simulink model "simulation_model"  (R2018b)
settings: Solver=ode45  StartTime=0.0  StopTime=20000  RelTol=1e-3
values from neighbouring files (symbols this model uses):
  DP = polyfit(CL_uav,CD_uav,2)    [intialize.m]
  Dprop = 0.482    [intialize.m]
  J = xlsread('UAVdata.xlsx','P3:P16')    [intialize.m]
  p0 = 0.03840634    [intialize.m]
  p1 = 0.04503419    [intialize.m]
  p2 = -0.06173971    [intialize.m]
  p3 = -0.06297906    [intialize.m]
  Sref = 0.6    [intialize.m]
  xx = [1000 1173.46938776 1346.93877551 1520.40816327 1693.87755102 1867.34693878 2040.81632653 2214.28571429 2387.75510204 2561.2244898 2734.69387755 2908.16326531 ... (50 elements, 1x50)]    [engine_data.mat]
  yy = [1.39285714286 1.7055393586 2.01822157434 2.33090379009 2.64358600583 2.95626822157 3.26895043732 3.58163265306 3.8943148688 4.20699708455 4.51967930029 4.83236151603 ... (50 elements, 1x50)]    [engine_data.mat]
  Zeng = [1318.54879102 1244.05943439 1169.57007776 1095.08072113 1020.59136451 950.389908425 918.779557259 887.169206094 855.558854928 823.948503763 795.179532477 777.776080712 ... (2500 elements, 50x50)]    [engine_data.mat]
settings Model: Creator=Rohith  LastModifiedBy=Rohith

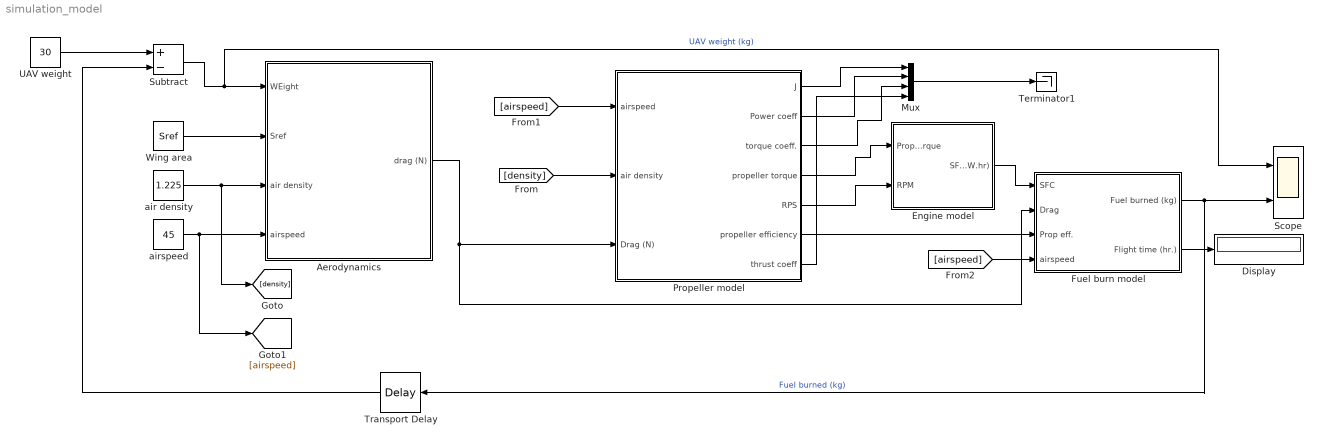
== system simulation_model ==
  Aerodynamics : Subsystem
  Display : Display
  Engine model : Subsystem
  Fuel burn model : Subsystem
  Mux : Mux
  Propeller model : Subsystem
  Scope : Scope  NumInputPorts=2
  Subtract : Sum  Inputs=+-
  Terminator1 : Terminator
  Transport Delay : TransportDelay  DelayTime=0.1
  UAV weight : Constant  Value=30
  Wing area : Constant  Value=Sref
  air density : Constant  Value=1.225
  airspeed : Constant  Value=45
  wires:
  Subtract/1 -> Scope/1, Aerodynamics/1(WEight)  "UAV weight (kg)"
  Wing area/1 -> Aerodynamics/2(Sref)
  air density/1 -> [density], Aerodynamics/3(air density)
  airspeed/1 -> [airspeed], Aerodynamics/4(airspeed)
  Aerodynamics/1(drag (N)) -> Propeller model/3(Drag (N)), Fuel burn model/2(Drag)
  [density] -> Propeller model/2(air density)
  [airspeed] -> Propeller model/1(airspeed)
  Propeller model/4(propeller torque) -> Engine model/1(Prop torque)
  Propeller model/5(RPS) -> Engine model/2(RPM)
  Engine model/1(SFC (kg/W.hr)) -> Fuel burn model/1(SFC)
  [airspeed] -> Fuel burn model/4(airspeed)
  Propeller model/6("propeller efficiency ") -> Fuel burn model/3(Prop eff.)
  Fuel burn model/1(Fuel burned (kg)) -> Scope/2, Transport Delay/1  "Fuel burned (kg)"
  Propeller model/1(J) -> Mux/1
  Propeller model/2(Power coeff) -> Mux/2
  Mux/1 -> Terminator1/1
  Propeller model/3(torque coeff.) -> Mux/3
  Propeller model/7(thrust coeff) -> Mux/4
  Fuel burn model/2(Flight time (hr.)) -> Display/1
  UAV weight/1 -> Subtract/1
  Transport Delay/1 -> Subtract/2

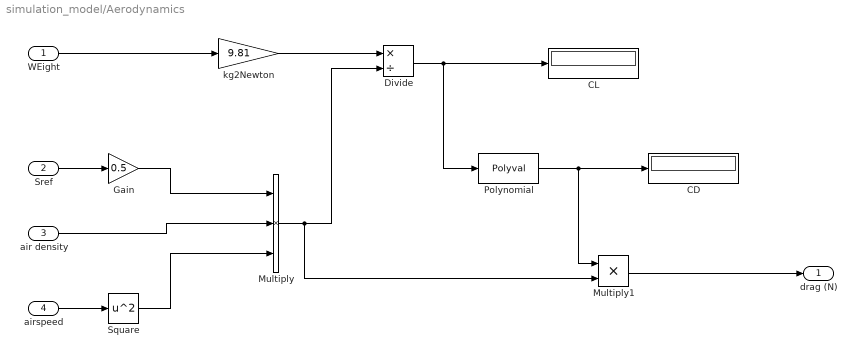
== system simulation_model/Aerodynamics ==
  WEight : Inport
  Sref : Inport  Port=2
  air density : Inport  Port=3
  airspeed : Inport  Port=4
  CD : Display
  CL : Display
  Divide : Product  Inputs=*/
  Gain : Gain  Gain=0.5
  Multiply : Product  Inputs=3
  Multiply1 : Product
  Polynomial : Polyval  Coefs="[DP(1)  DP(2)  DP(3)]"
  Square : Math  Operator=square  SaturateOnIntegerOverflow=on
  kg2Newton : Gain  Gain=9.81
  drag (N) : Outport
  wires:
  Sref/1 -> Gain/1
  Divide/1 -> Polynomial/1, CL/1
  Multiply1/1 -> drag (N)/1
  Square/1 -> Multiply/3
  Polynomial/1 -> Multiply1/1, CD/1
  kg2Newton/1 -> Divide/1
  Gain/1 -> Multiply/1
  Multiply/1 -> Multiply1/2, Divide/2
  WEight/1 -> kg2Newton/1
  airspeed/1 -> Square/1
  air density/1 -> Multiply/2

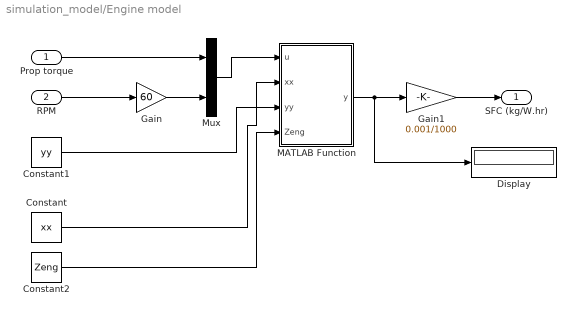
== system simulation_model/Engine model ==
  Prop torque : Inport
  RPM : Inport  Port=2
  Constant : Constant  Value=xx
  Constant1 : Constant  Value=yy
  Constant2 : Constant  Value=Zeng
  Display : Display
  Gain : Gain  Gain=60
  Gain1 : Gain  Gain=0.001/1000
  MATLAB Function : MATLAB Function  TreatAsAtomicUnit=on
  Mux : Mux  Inputs=2
  SFC (kg/W.hr) : Outport
  wires:
  RPM/1 -> Gain/1
  Prop torque/1 -> Mux/1
  Mux/1 -> MATLAB Function/1(u)
  MATLAB Function/1(y) -> Display/1, Gain1/1
  Constant/1 -> MATLAB Function/2(xx)
  Constant1/1 -> MATLAB Function/3(yy)
  Constant2/1 -> MATLAB Function/4(Zeng)
  Gain/1 -> Mux/2
  Gain1/1 -> SFC (kg/W.hr)/1

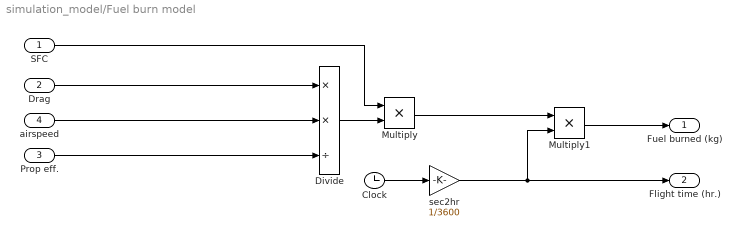
== system simulation_model/Fuel burn model ==
  SFC : Inport
  Drag : Inport  Port=2
  Prop eff. : Inport  Port=3
  airspeed : Inport  Port=4
  Clock : Clock
  Divide : Product  Inputs=**/
  Multiply : Product
  Multiply1 : Product
  sec2hr : Gain  Gain=1/3600
  Fuel burned (kg) : Outport
  Flight time (hr.) : Outport  Port=2
  wires:
  airspeed/1 -> Divide/2
  Prop eff./1 -> Divide/3
  Divide/1 -> Multiply/2
  SFC/1 -> Multiply/1
  Multiply/1 -> Multiply1/1
  Clock/1 -> sec2hr/1
  sec2hr/1 -> Flight time (hr.)/1, Multiply1/2
  Drag/1 -> Divide/1
  Multiply1/1 -> Fuel burned (kg)/1

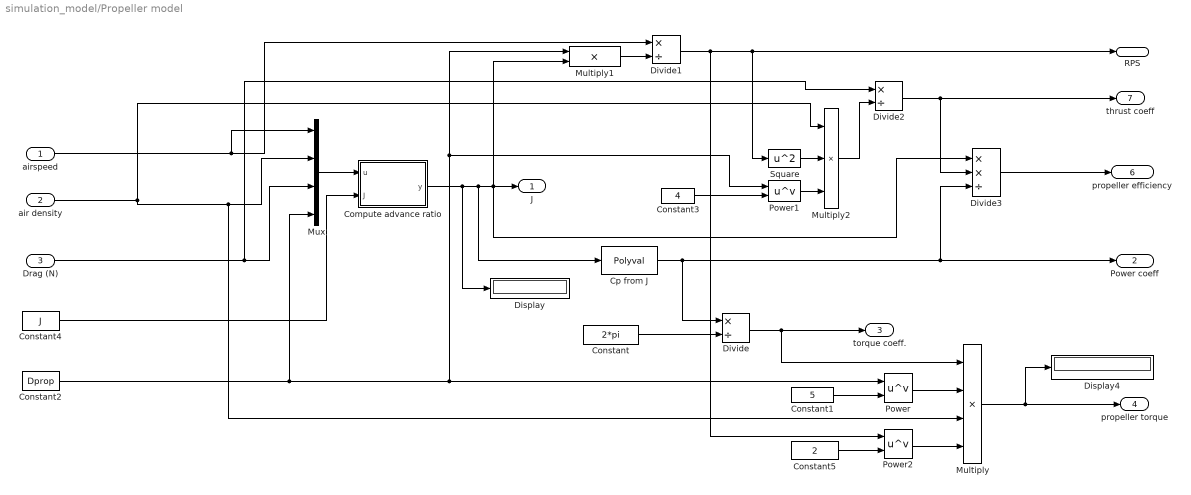
== system simulation_model/Propeller model ==
  airspeed : Inport
  air density : Inport  Port=2
  Drag (N) : Inport  Port=3
  Compute advance ratio : MATLAB Function  TreatAsAtomicUnit=on
  Constant : Constant  Value=2*pi
  Constant1 : Constant  Value=5
  Constant2 : Constant  Value=Dprop
  Constant3 : Constant  Value=4
  Constant4 : Constant  Value=J  VectorParams1D=off
  Constant5 : Constant  Value=2
  Cp from J : Polyval  Coefs=[p3 p2 p1 p0]
  Display : Display
  Display4 : Display
  Divide : Product  Inputs=*/
  Divide1 : Product  Inputs=*/
  Divide2 : Product  Inputs=*/
  Divide3 : Product  Inputs=**/
  Multiply : Product  Inputs=4
  Multiply1 : Product
  Multiply2 : Product  Inputs=3
  Mux : Mux
  Power : Math  Operator=pow  SaturateOnIntegerOverflow=on
  Power1 : Math  Operator=pow  SaturateOnIntegerOverflow=on
  Power2 : Math  Operator=pow  SaturateOnIntegerOverflow=on
  Square : Math  Operator=square  SaturateOnIntegerOverflow=on
  J : Outport
  Power coeff : Outport  Port=2
  torque coeff. : Outport  Port=3
  propeller torque : Outport  Port=4
  RPS : Outport  Port=5
  "propeller efficiency " : Outport  Port=6
  thrust coeff : Outport  Port=7
  wires:
  Mux/1 -> Compute advance ratio/1(u)
  airspeed/1 -> Divide1/1, Mux/1
  Compute advance ratio/1(y) -> Display/1, Cp from J/1, J/1, Divide3/1, Multiply1/2
  Drag (N)/1 -> Divide2/1, Mux/3
  Cp from J/1 -> Divide/1, Divide3/3, Power coeff/1
  Constant/1 -> Divide/2
  Divide/1 -> Multiply/1, torque coeff./1
  Multiply/1 -> Display4/1, propeller torque/1
  air density/1 -> Multiply/3, Mux/2, Multiply2/1
  Constant1/1 -> Power/2
  Power/1 -> Multiply/2
  Divide1/1 -> Power2/1, Square/1, RPS/1
  Multiply1/1 -> Divide1/2
  Divide2/1 -> Divide3/2, thrust coeff/1
  Multiply2/1 -> Divide2/2
  Square/1 -> Multiply2/2
  Power1/1 -> Multiply2/3
  Constant3/1 -> Power1/2
  Divide3/1 -> "propeller efficiency "/1
  Constant4/1 -> Compute advance ratio/2(J)
  Constant2/1 -> Multiply1/1, Power1/1, Power/1, Mux/4
  Power2/1 -> Multiply/4
  Constant5/1 -> Power2/2

== matlab function simulation_model/Engine model/MATLAB Function ==
  data: u input; xx input; yy input; y output; Zeng input
function y = fcn(u,xx,yy,Zeng)
%#codegen
torque=u(1);
RPM=u(2);


SFC=interp2(xx,yy,Zeng,RPM,torque);
SFC(isnan(SFC))=2700;
y = SFC;

== matlab function simulation_model/Propeller model/Compute advance ratio ==
  data: u input; y output; J input
function y = fcn(u,J)
%#codegen
V=u(1);
rho=u(2);
Drag=u(3);
Dprop=u(4);

% rotations per second
rps_J=V.*(J.*Dprop).^-1; 

% compute advance ratio from data
J2=V*(rps_J*Dprop).^-1; 

% thrust coeff. from advance ratio
Ct=(0.05017951*J2.^3)-(0.1638384*J2.^2)-(0.03857363*J2)+0.1079442; 

% compute thrust to be produced by the propeller in N
Tprop=(Ct*rho.*rps_J.^2*Dprop.^4);
TJ=polyfit(Tprop,J2,3);

%operating advance ratio
J_req=TJ(1)*Drag.^3+TJ(2)*Drag.^2+TJ(3)*Drag+TJ(4);


y =J_req;
